simulink model "aufgabe6_sim"  (R2017b)
settings: Solver=VariableStepAuto  StartTime=0.0  StopTime=1  RelTol=1e-3
values from neighbouring files (symbols this model uses):
  Cr = ((km*i)-Mm(:,4))./W(:,4)    [aufgabe2_cr.m]    (also in aufgabe3.m = 5e-06; aufgabe4.m = 5e-06; aufgabe6.m = 5e-06)
  J = 0.5e-6    (= 5e-07)    [aufgabe3.m]    (also in aufgabe4.m = 3e-06; aufgabe6.m = 3e-06)
  ke = 0.024    [aufgabe2_cr.m]    (also in aufgabe3.m; aufgabe4.m; aufgabe6.m)
  ki = (J*R)/km * w0^2    (= 5.6347826087)    [aufgabe6.m]
  km = 0.0232    [aufgabe2_cr.m]    (also in aufgabe3.m = 0.0227; aufgabe4.m = 0.023; aufgabe6.m = 0.023)
  kp = 1/km * (2*D*w0*J*R-ke*km-Cr*R)    (= 0.0204260869565)    [aufgabe6.m]
  L = Lm+Ls    [aufgabe2.m]    (also in aufgabe2_cr.m = 0.0004; aufgabe3.m = 0.0004; aufgabe4.m = 0.0004; aufgabe6.m = 0.0004)
  Ml = 0    [aufgabe2_cr.m]    (also in aufgabe3.m; aufgabe6.m)
  R = 3+(2*rand-1)*0.4    [aufgabe1.m]    (also in aufgabe2.m = 3; aufgabe2_cr.m = 3; aufgabe3.m = 3; aufgabe4.m = 3)
settings Model: Creator=gurbuz  LastModifiedBy=gurbuz

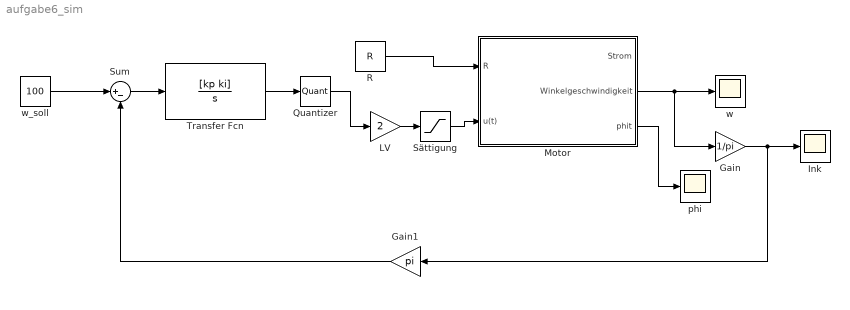
== system aufgabe6_sim ==
  Gain : Gain  Gain=1/pi
  Gain1 : Gain  Gain=pi
  Ink : Scope
  LV : Gain  Gain=2
  "Motor " : Subsystem
  Quantizer : Quantizer  QuantizationInterval=20/2^16
  R : Constant  Value=R
  Sum : Sum  Inputs=|+-
  Sättigung : Saturate  UpperLimit=12  LowerLimit=-12
  Transfer Fcn : TransferFcn  Numerator=[kp ki]  Denominator=[1 0]
  phi : Scope
  "w " : Scope
  "w_soll " : Constant  Value=100
  wires:
  "w_soll "/1 -> Sum/1
  "Motor "/2(Winkelgeschwindigkeit) -> Gain/1, "w "/1
  "Motor "/3("phit ") -> phi/1
  Gain/1 -> Gain1/1, Ink/1
  Gain1/1 -> Sum/2
  Quantizer/1 -> LV/1
  R/1 -> "Motor "/1("R ")
  LV/1 -> Sättigung/1
  Sättigung/1 -> "Motor "/2(u(t))
  Sum/1 -> Transfer Fcn/1
  Transfer Fcn/1 -> Quantizer/1

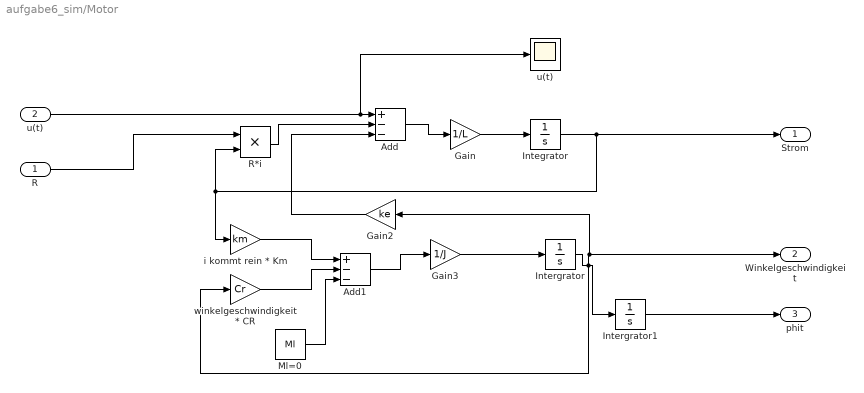
== system aufgabe6_sim/Motor  ==
  "R " : Inport
  u(t) : Inport  Port=2
  Add : Sum  Inputs=+--
  Add1 : Sum  Inputs=+--
  Gain : Gain  Gain=1/L
  Gain2 : Gain  Gain=ke
  Gain3 : Gain  Gain=1/J
  Integrator : Integrator
  Intergrator : Integrator
  Intergrator1 : Integrator
  "Ml=0 " : Constant  Value=Ml
  R*i : Product
  "i kommt rein * Km " : Gain  Gain=km
  "u(t) " : Scope
  "winkelgeschwindigkeit * CR " : Gain  Gain=Cr
  Strom : Outport
  Winkelgeschwindigkeit : Outport  Port=2
  "phit " : Outport  Port=3
  wires:
  Gain/1 -> Integrator/1
  Add/1 -> Gain/1
  Gain3/1 -> Intergrator/1
  u(t)/1 -> "u(t) "/1, Add/1
  "winkelgeschwindigkeit * CR "/1 -> Add1/2
  Integrator/1 -> Strom/1, R*i/2, "i kommt rein * Km "/1
  R*i/1 -> Add/2
  Intergrator/1 -> Intergrator1/1, "winkelgeschwindigkeit * CR "/1, Winkelgeschwindigkeit/1, Gain2/1
  Gain2/1 -> Add/3
  Add1/1 -> Gain3/1
  "Ml=0 "/1 -> Add1/3
  "i kommt rein * Km "/1 -> Add1/1
  Intergrator1/1 -> "phit "/1
  "R "/1 -> R*i/1
